simulink model "bench_aux"  (R2024b)
settings: Solver=daessc  StartTime=0.0  StopTime=10  MaxStep=1e-2  RelTol=1e-3
libraries: loco_native_lib x2, fl_lib x1, nesl_utility x1
settings Model: Creator=BillBeverley  LastModifiedBy=BillBeverley

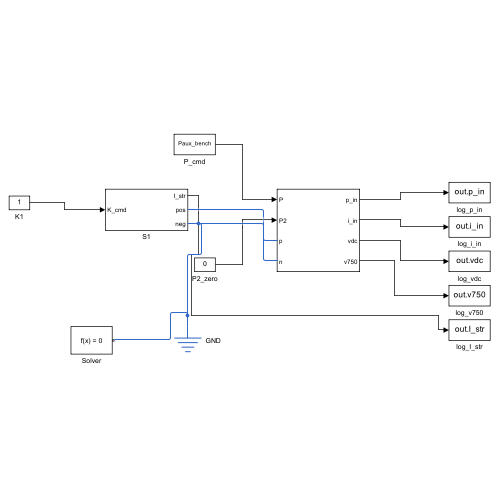
[thumbnail: Simulink's stored preview of the top-level diagram]
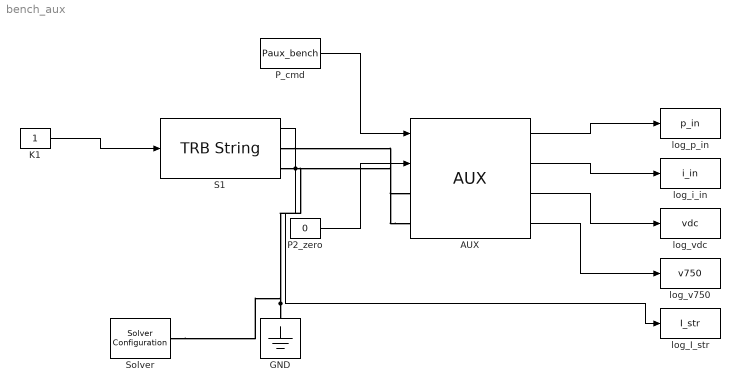
== system bench_aux ==
  AUX : loco_native_lib/AUX  eta=P.aux.eta  P_max=P.aux.P_max  V750=750  V_floor=100
  GND : fl_lib/Electrical/Electrical Elements/Electrical Reference
  K1 : Constant
  P2_zero : Constant  Value=0
  P_cmd : FromWorkspace  VariableName=Paux_bench
  S1 : loco_native_lib/TRB String  SystemSampleTime=-1  VariantActivationTime=update diagram  AllowFlexibleInterface=on  Latency=0  AutoFrameSizeCalculation=off
  Solver : nesl_utility/Solver Configuration  PhysicalDomain=network_engine_domain  SubClassName=solver  LeftPortType=input  RightPortType=generic  Tones=[]  Harmonics=[]  SimulateNoise=off  Profile=off  UseLocalSampling=off  EnableSwitchedLinearOptims=on  FrequencyDomain=off  UseCCode=off  RelTol=0.001  AbsTol=0.001  MinStep=1e-09  ToWorkspace=off  RevertToSquareIcSolve=off  NumHomotopyIterations=100  PhasorMode=off  PhasorModeNumHarmonics=1  ConsistencySolver=NEWTON_XTOL_AFTER_FTOL  IndexReductionMethod=DerivativeReplacement  DoDC=off  ResidualTolerance=1e-09  ConsistencyTolSource=GLOBAL  ConsistencyAbsTol=0.001  ConsistencyRelTol=0.001  ConsistencyTolFactor=0.001  UseLocalSolver=off  LocalSolverChoice=NE_BACKWARD_EULER_ADVANCER  ResolveIndetEquations=on  FunctionEvalNumThread=1  LocalSolverSampleTime=0.001  DoFixedCost=off  MaxNonlinIter=3  MaxModeIter=2  ComputeImpulses=off  ImpulseIterations=2  LinearAlgebra=auto  LinearAlgebraNumThread=0  EquationFormulation=NE_TIME_EF  DelaysMemoryBudget=1024  AutomaticFiltering=on  FilteringTimeConstant=0.001  PartitionStorageMethod=AS_NEEDED  PartitionMemoryBudget=1024  PartitionMethod=ROBUST  MultibodyUseLocalSolver=off  MultibodyLocalSolverChoice=ODE1  MultibodyLocalSolverSampleTime=0.001
  log_I_str : ToWorkspace  VariableName=I_str  SaveFormat=Timeseries  SampleTime=-1
  log_i_in : ToWorkspace  VariableName=i_in  SaveFormat=Timeseries  SampleTime=-1
  log_p_in : ToWorkspace  VariableName=p_in  SaveFormat=Timeseries  SampleTime=-1
  log_v750 : ToWorkspace  VariableName=v750  SaveFormat=Timeseries  SampleTime=-1
  log_vdc : ToWorkspace  VariableName=vdc  SaveFormat=Timeseries  SampleTime=-1
  wires:
  K1/1 -> S1/1
  P_cmd/1 -> AUX/1
  P2_zero/1 -> AUX/2
  AUX/1 -> log_p_in/1
  AUX/2 -> log_i_in/1
  AUX/3 -> log_vdc/1
  AUX/4 -> log_v750/1
  S1/1 -> log_I_str/1
  connections:
  S1/RConn1 -- AUX/LConn1
  AUX/LConn2 -- S1/RConn2 -- GND/LConn1 -- Solver/RConn1
